simulink model "nnSystem"  (R2024b)
settings: Solver=FixedStepAuto  StartTime=0.0  StopTime=10.0  RelTol=1e-3
undefined symbols (not defined in the file or in its folder): tnet
libraries: dlconvfclib x15, dlutilitylib x6, dlcombinationlib x5, dlactivationlib x2
settings Model: Creator=bzhuang  LastModifiedBy=bzhuang
settings OptimizationCC: DefaultParameterBehavior=Inlined  EnhancedBackFolding=on  PassReuseOutputArgsAs=Individual arguments  ZeroExternalMemoryAtStartup=off  ZeroInternalMemoryAtStartup=off  OptimizeBlockOrder=speed  DifferentSizesBufferReuse=on  OptimizationCustomize=off  EfficientTunableParamExpr=on
settings DebuggingCC: ParameterTunabilityLossMsg=error
settings SFSimCC: MATLABDynamicMemAlloc=off
settings RTWCC: Description=Embedded Coder  SystemTargetFile=ert.tlc  TemplateMakefile=ert_default_tmf
settings CodeAppCC: ForceParamTrailComments=on  IgnoreCustomStorageClasses=off  OperatorAnnotations=on  SimulinkDataObjDesc=on  SFDataObjDesc=on  InsertBlockDesc=on
settings ERTTargetCC: TargetLangStandard=C99 (ISO)  GenerateSampleERTMain=on  ERTCustomFileTemplate=example_file_process.tlc

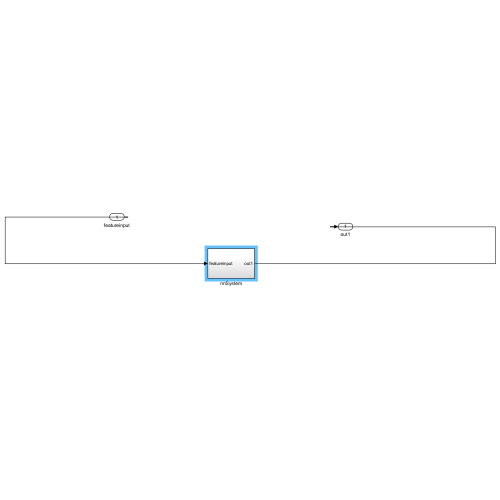
[thumbnail: Simulink's stored preview of the top-level diagram]
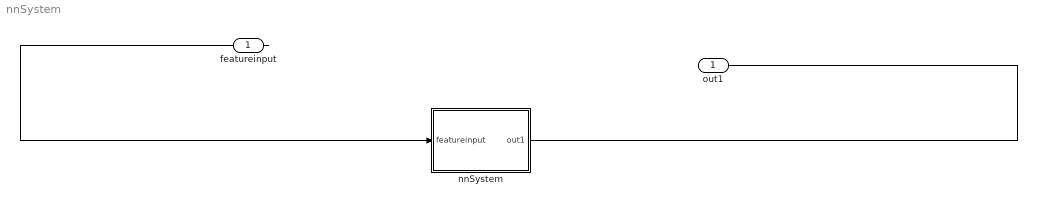
== system nnSystem ==
  featureinput : Inport  PortDimensions=[3]
  nnSystem : Subsystem
  out1 : Outport
  wires:
  featureinput/1 -> nnSystem/1(featureinput)
  nnSystem/1(out1) -> out1/1

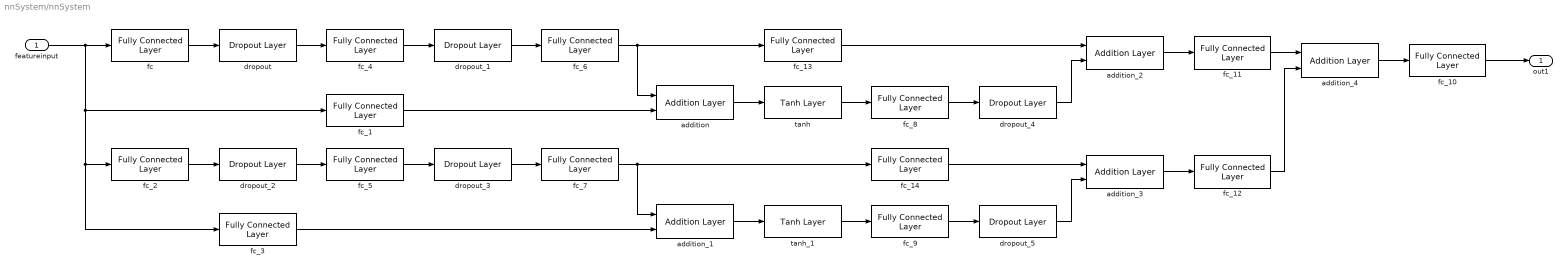
== system nnSystem/nnSystem ==
  featureinput : Inport  PortDimensions=[3]
  addition : dlcombinationlib/Addition Layer  NumInputs=2  OutMin=[]  OutMax=[]  SampleTime=-1
      settings: DataFormat=C
  addition_{1..4} (4 alike) : dlcombinationlib/Addition Layer  NumInputs=2  OutMin=[]  OutMax=[]  SampleTime=-1
      settings: DataFormat=C
  dropout : dlutilitylib/Dropout Layer  SampleTime=-1
  dropout_{1..5} (5 alike) : dlutilitylib/Dropout Layer  SampleTime=-1
  fc : dlconvfclib/Fully Connected Layer  Layer=tnet.Layers(2)  OutMin=[]  OutMax=[]  WeightsDataTypeStr=Inherit: Inherit via back propagation  WeightsMin=[]  WeightsMax=[]  BiasDataTypeStr=Inherit: Inherit via back propagation  BiasMin=[]  BiasMax=[]  MatrixMultiplyMin=[]  MatrixMultiplyMax=[]  SampleTime=-1
      settings: DataFormat=C
  fc_1 : dlconvfclib/Fully Connected Layer  Layer=tnet.Layers(7)  OutMin=[]  OutMax=[]  WeightsDataTypeStr=Inherit: Inherit via back propagation  WeightsMin=[]  WeightsMax=[]  BiasDataTypeStr=Inherit: Inherit via back propagation  BiasMin=[]  BiasMax=[]  MatrixMultiplyMin=[]  MatrixMultiplyMax=[]  SampleTime=-1
      settings: DataFormat=C
  fc_10 : dlconvfclib/Fully Connected Layer  Layer=tnet.Layers(29)  OutMin=[]  OutMax=[]  WeightsDataTypeStr=Inherit: Inherit via back propagation  WeightsMin=[]  WeightsMax=[]  BiasDataTypeStr=Inherit: Inherit via back propagation  BiasMin=[]  BiasMax=[]  MatrixMultiplyMin=[]  MatrixMultiplyMax=[]  SampleTime=-1
      settings: DataFormat=C
  fc_11 : dlconvfclib/Fully Connected Layer  Layer=tnet.Layers(25)  OutMin=[]  OutMax=[]  WeightsDataTypeStr=Inherit: Inherit via back propagation  WeightsMin=[]  WeightsMax=[]  BiasDataTypeStr=Inherit: Inherit via back propagation  BiasMin=[]  BiasMax=[]  MatrixMultiplyMin=[]  MatrixMultiplyMax=[]  SampleTime=-1
      settings: DataFormat=C
  fc_12 : dlconvfclib/Fully Connected Layer  Layer=tnet.Layers(27)  OutMin=[]  OutMax=[]  WeightsDataTypeStr=Inherit: Inherit via back propagation  WeightsMin=[]  WeightsMax=[]  BiasDataTypeStr=Inherit: Inherit via back propagation  BiasMin=[]  BiasMax=[]  MatrixMultiplyMin=[]  MatrixMultiplyMax=[]  SampleTime=-1
      settings: DataFormat=C
  fc_13 : dlconvfclib/Fully Connected Layer  Layer=tnet.Layers(18)  OutMin=[]  OutMax=[]  WeightsDataTypeStr=Inherit: Inherit via back propagation  WeightsMin=[]  WeightsMax=[]  BiasDataTypeStr=Inherit: Inherit via back propagation  BiasMin=[]  BiasMax=[]  MatrixMultiplyMin=[]  MatrixMultiplyMax=[]  SampleTime=-1
      settings: DataFormat=C
  fc_14 : dlconvfclib/Fully Connected Layer  Layer=tnet.Layers(23)  OutMin=[]  OutMax=[]  WeightsDataTypeStr=Inherit: Inherit via back propagation  WeightsMin=[]  WeightsMax=[]  BiasDataTypeStr=Inherit: Inherit via back propagation  BiasMin=[]  BiasMax=[]  MatrixMultiplyMin=[]  MatrixMultiplyMax=[]  SampleTime=-1
      settings: DataFormat=C
  fc_2 : dlconvfclib/Fully Connected Layer  Layer=tnet.Layers(8)  OutMin=[]  OutMax=[]  WeightsDataTypeStr=Inherit: Inherit via back propagation  WeightsMin=[]  WeightsMax=[]  BiasDataTypeStr=Inherit: Inherit via back propagation  BiasMin=[]  BiasMax=[]  MatrixMultiplyMin=[]  MatrixMultiplyMax=[]  SampleTime=-1
      settings: DataFormat=C
  fc_3 : dlconvfclib/Fully Connected Layer  Layer=tnet.Layers(13)  OutMin=[]  OutMax=[]  WeightsDataTypeStr=Inherit: Inherit via back propagation  WeightsMin=[]  WeightsMax=[]  BiasDataTypeStr=Inherit: Inherit via back propagation  BiasMin=[]  BiasMax=[]  MatrixMultiplyMin=[]  MatrixMultiplyMax=[]  SampleTime=-1
      settings: DataFormat=C
  fc_4 : dlconvfclib/Fully Connected Layer  Layer=tnet.Layers(4)  OutMin=[]  OutMax=[]  WeightsDataTypeStr=Inherit: Inherit via back propagation  WeightsMin=[]  WeightsMax=[]  BiasDataTypeStr=Inherit: Inherit via back propagation  BiasMin=[]  BiasMax=[]  MatrixMultiplyMin=[]  MatrixMultiplyMax=[]  SampleTime=-1
      settings: DataFormat=C
  fc_5 : dlconvfclib/Fully Connected Layer  Layer=tnet.Layers(10)  OutMin=[]  OutMax=[]  WeightsDataTypeStr=Inherit: Inherit via back propagation  WeightsMin=[]  WeightsMax=[]  BiasDataTypeStr=Inherit: Inherit via back propagation  BiasMin=[]  BiasMax=[]  MatrixMultiplyMin=[]  MatrixMultiplyMax=[]  SampleTime=-1
      settings: DataFormat=C
  fc_6 : dlconvfclib/Fully Connected Layer  Layer=tnet.Layers(6)  OutMin=[]  OutMax=[]  WeightsDataTypeStr=Inherit: Inherit via back propagation  WeightsMin=[]  WeightsMax=[]  BiasDataTypeStr=Inherit: Inherit via back propagation  BiasMin=[]  BiasMax=[]  MatrixMultiplyMin=[]  MatrixMultiplyMax=[]  SampleTime=-1
      settings: DataFormat=C
  fc_7 : dlconvfclib/Fully Connected Layer  Layer=tnet.Layers(12)  OutMin=[]  OutMax=[]  WeightsDataTypeStr=Inherit: Inherit via back propagation  WeightsMin=[]  WeightsMax=[]  BiasDataTypeStr=Inherit: Inherit via back propagation  BiasMin=[]  BiasMax=[]  MatrixMultiplyMin=[]  MatrixMultiplyMax=[]  SampleTime=-1
      settings: DataFormat=C
  fc_8 : dlconvfclib/Fully Connected Layer  Layer=tnet.Layers(16)  OutMin=[]  OutMax=[]  WeightsDataTypeStr=Inherit: Inherit via back propagation  WeightsMin=[]  WeightsMax=[]  BiasDataTypeStr=Inherit: Inherit via back propagation  BiasMin=[]  BiasMax=[]  MatrixMultiplyMin=[]  MatrixMultiplyMax=[]  SampleTime=-1
      settings: DataFormat=C
  fc_9 : dlconvfclib/Fully Connected Layer  Layer=tnet.Layers(21)  OutMin=[]  OutMax=[]  WeightsDataTypeStr=Inherit: Inherit via back propagation  WeightsMin=[]  WeightsMax=[]  BiasDataTypeStr=Inherit: Inherit via back propagation  BiasMin=[]  BiasMax=[]  MatrixMultiplyMin=[]  MatrixMultiplyMax=[]  SampleTime=-1
      settings: DataFormat=C
  tanh : dlactivationlib/Tanh Layer  ApproximationMethod=None  SampleTime=-1
  tanh_1 : dlactivationlib/Tanh Layer  ApproximationMethod=None  SampleTime=-1
  out1 : Outport
  wires:
  fc_12/1 -> addition_4/2
  fc_1/1 -> addition/2
  addition/1 -> tanh/1
  fc_8/1 -> dropout_4/1
  featureinput/1 -> fc_3/1, fc_2/1, fc_1/1, fc/1
  fc_3/1 -> addition_1/2
  fc_6/1 -> fc_13/1, addition/1
  tanh_1/1 -> fc_9/1
  fc_7/1 -> fc_14/1, addition_1/1
  dropout_1/1 -> fc_6/1
  dropout_4/1 -> addition_2/2
  fc_11/1 -> addition_4/1
  dropout_3/1 -> fc_7/1
  addition_4/1 -> fc_10/1
  fc_4/1 -> dropout_1/1
  dropout_5/1 -> addition_3/2
  fc/1 -> dropout/1
  fc_14/1 -> addition_3/1
  fc_13/1 -> addition_2/1
  addition_3/1 -> fc_12/1
  addition_2/1 -> fc_11/1
  fc_2/1 -> dropout_2/1
  tanh/1 -> fc_8/1
  fc_9/1 -> dropout_5/1
  dropout_2/1 -> fc_5/1
  addition_1/1 -> tanh_1/1
  fc_10/1 -> out1/1
  fc_5/1 -> dropout_3/1
  dropout/1 -> fc_4/1
